simulink model "ue_1_b"  (R2015b)
settings: Solver=VariableStepAuto  StartTime=0.0  StopTime=500  RelTol=1e-3
settings Model: Creator=dbarelop  LastModifiedBy=Admin

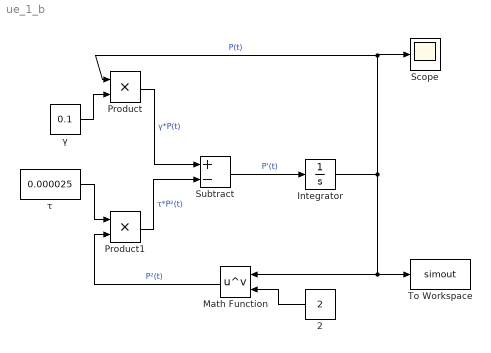
== system ue_1_b ==
  " τ" : Constant  Value=0.000025
  2 : Constant  Value=2
  Integrator : Integrator  InitialCondition=10000
  Math Function : Math  Operator=pow  OutputSignalType=real  SaturateOnIntegerOverflow=on
  Product : Product
  Product1 : Product
  Scope : Scope
  Subtract : Sum  Inputs=+-
  To Workspace : ToWorkspace  VariableName=simout  SaveFormat=Timeseries  SampleTime=-1
  γ : Constant  Value=0.1
  wires:
  Subtract/1 -> Integrator/1  "P'(t)"
  Integrator/1 -> Scope/1, Product/1, Math Function/1, To Workspace/1  "P(t)"
  Product/1 -> Subtract/1  "γ*P(t)"
  γ/1 -> Product/2
  " τ"/1 -> Product1/1
  Math Function/1 -> Product1/2  "P²(t)"
  Product1/1 -> Subtract/2  "τ*P²(t)"
  2/1 -> Math Function/2
